simulink model "ThreePhTrans"  (R2020b)
settings: Solver=ode23t  StartTime=0.0  StopTime=0.2  RelTol=1e-3
libraries: powerlib x32
settings Model: Creator=ashka  LastModifiedBy=ashka

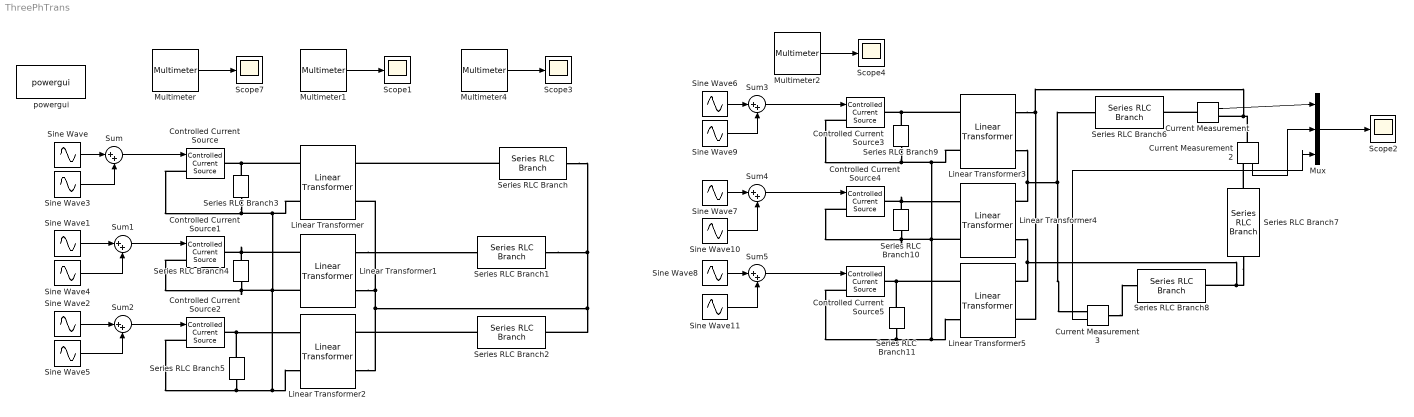
== system ThreePhTrans ==
  Controlled Current Source{,1..5} (6 alike) : powerlib/Electrical Sources/Controlled Current Source  Initialize=on  Source_Type=AC  Amplitude=0  Phase=0  Frequency=0  Measurements=Current
  Current Measurement : powerlib/Measurements/Current Measurement  PhasorSimulation=off  OutputType=Complex  PSBequivalent=0
  Current Measurement2 : powerlib/Measurements/Current Measurement  PhasorSimulation=off  OutputType=Complex  PSBequivalent=0
  Current Measurement3 : powerlib/Measurements/Current Measurement  PhasorSimulation=off  OutputType=Complex  PSBequivalent=0
  Linear Transformer{,1..5} (6 alike) : powerlib/Elements/Linear Transformer  UNITS=SI  NominalPower=[ 10e3 50 ]  winding1=[400 2 0.45856]  winding2=[4000 0.7938 0.084225]  ThreeWindings=off  winding3=[3.15e+05 0.7938 0.084225]  RmLm=[1.0805e+06 2866]  Measurements=None  DataType=on
  Multimeter : powerlib/Measurements/Multimeter  Tag=PoWeRsYsTeMmEaSuReMeNt  PhasorSimulation=off  OutputType=Magnitude  sel=[10 11 12]  L=15  Gain=[1 1 1]  yselected={'Isrc: Controlled Current Source','Isrc: Controlled Current Source1','Isrc: Controlled Current Source2'};  PSBOutputType=1  PSBequivalent=0  AxesSetting=[0,0.1,-100,100]  Display=0  SavedBlockNames=-11
      settings: AttributesFormatString=\n
  Multimeter1 : powerlib/Measurements/Multimeter  Tag=PoWeRsYsTeMmEaSuReMeNt  PhasorSimulation=off  OutputType=Magnitude  sel=[7 8 9]  L=15  Gain=[1 1 1]  yselected={'Ib: Series RLC Branch','Ib: Series RLC Branch1','Ib: Series RLC Branch2'};  PSBOutputType=1  PSBequivalent=0  AxesSetting=[0,0.1,-100,100]  Display=0  SavedBlockNames=-11
      settings: AttributesFormatString=\n
  Multimeter2 : powerlib/Measurements/Multimeter  Tag=PoWeRsYsTeMmEaSuReMeNt  PhasorSimulation=off  OutputType=Magnitude  sel=[13 14 15]  L=15  Gain=[1 1 1]  yselected={'Isrc: Controlled Current Source3','Isrc: Controlled Current Source4','Isrc: Controlled Current Source5'};  PSBOutputType=1  PSBequivalent=0  AxesSetting=[0,0.1,-100,100]  Display=0  SavedBlockNames=-11
      settings: AttributesFormatString=\n
  Multimeter4 : powerlib/Measurements/Multimeter  Tag=PoWeRsYsTeMmEaSuReMeNt  PhasorSimulation=off  OutputType=Magnitude  sel=[1 2 5]  L=15  Gain=[1 1 1]  yselected={'Ub: Series RLC Branch','Ub: Series RLC Branch1','Ub: Series RLC Branch2'};  PSBOutputType=1  PSBequivalent=0  AxesSetting=[0,0.1,-100,100]  Display=0  SavedBlockNames=-11
      settings: AttributesFormatString=\n
  Mux : Mux  Inputs=3
  Scope{1..4,7} (5 alike) : Scope
  Series RLC Branch : powerlib/Elements/Series RLC Branch  LConnTagsString=__new0  RConnTagsString=__new0  BranchType=R  Resistance=100  Inductance=1e-3  SetiL0=off  InitialCurrent=0  Capacitance=1e-6  Setx0=off  InitialVoltage=0  Measurements=Branch voltage and current
  Series RLC Branch1 : powerlib/Elements/Series RLC Branch  LConnTagsString=__new0  RConnTagsString=__new0  BranchType=R  Resistance=100  Inductance=1e-3  SetiL0=off  InitialCurrent=0  Capacitance=1e-6  Setx0=off  InitialVoltage=0  Measurements=Branch voltage and current
  Series RLC Branch10 : powerlib/Elements/Series RLC Branch  LConnTagsString=__new0  RConnTagsString=__new0  BranchType=R  Resistance=1e6  Inductance=1e-3  SetiL0=off  InitialCurrent=0  Capacitance=1e-6  Setx0=off  InitialVoltage=0  Measurements=Branch voltage
  Series RLC Branch11 : powerlib/Elements/Series RLC Branch  LConnTagsString=__new0  RConnTagsString=__new0  BranchType=R  Resistance=1e6  Inductance=1e-3  SetiL0=off  InitialCurrent=0  Capacitance=1e-6  Setx0=off  InitialVoltage=0  Measurements=Branch voltage
  Series RLC Branch2 : powerlib/Elements/Series RLC Branch  LConnTagsString=__new0  RConnTagsString=__new0  BranchType=R  Resistance=100  Inductance=1e-3  SetiL0=off  InitialCurrent=0  Capacitance=1e-6  Setx0=off  InitialVoltage=0  Measurements=Branch voltage and current
  Series RLC Branch3 : powerlib/Elements/Series RLC Branch  LConnTagsString=__new0  RConnTagsString=__new0  BranchType=R  Resistance=1e6  Inductance=1e-3  SetiL0=off  InitialCurrent=0  Capacitance=1e-6  Setx0=off  InitialVoltage=0  Measurements=None
  Series RLC Branch4 : powerlib/Elements/Series RLC Branch  LConnTagsString=__new0  RConnTagsString=__new0  BranchType=R  Resistance=1e6  Inductance=1e-3  SetiL0=off  InitialCurrent=0  Capacitance=1e-6  Setx0=off  InitialVoltage=0  Measurements=None
  Series RLC Branch5 : powerlib/Elements/Series RLC Branch  LConnTagsString=__new0  RConnTagsString=__new0  BranchType=R  Resistance=1e6  Inductance=1e-3  SetiL0=off  InitialCurrent=0  Capacitance=1e-6  Setx0=off  InitialVoltage=0  Measurements=None
  Series RLC Branch6 : powerlib/Elements/Series RLC Branch  LConnTagsString=__new0  RConnTagsString=__new0  BranchType=R  Resistance=100  Inductance=1e-3  SetiL0=off  InitialCurrent=0  Capacitance=1e-6  Setx0=off  InitialVoltage=0  Measurements=None
  Series RLC Branch7 : powerlib/Elements/Series RLC Branch  LConnTagsString=__new0  RConnTagsString=__new0  BranchType=R  Resistance=100  Inductance=1e-3  SetiL0=off  InitialCurrent=0  Capacitance=1e-6  Setx0=off  InitialVoltage=0  Measurements=None
  Series RLC Branch8 : powerlib/Elements/Series RLC Branch  LConnTagsString=__new0  RConnTagsString=__new0  BranchType=R  Resistance=100  Inductance=1e-3  SetiL0=off  InitialCurrent=0  Capacitance=1e-6  Setx0=off  InitialVoltage=0  Measurements=None
  Series RLC Branch9 : powerlib/Elements/Series RLC Branch  LConnTagsString=__new0  RConnTagsString=__new0  BranchType=R  Resistance=1e6  Inductance=1e-3  SetiL0=off  InitialCurrent=0  Capacitance=1e-6  Setx0=off  InitialVoltage=0  Measurements=Branch voltage
  Sine Wave : Sin  Amplitude=40  Frequency=2*pi*50  SampleTime=0
  Sine Wave1 : Sin  Amplitude=40  Frequency=2*pi*50  Phase=120*pi/180  SampleTime=0
  Sine Wave10 : Sin  Amplitude=10  Frequency=2*pi*150  Phase=120*pi/180*30  SampleTime=0
  Sine Wave11 : Sin  Amplitude=10  Frequency=2*pi*150  Phase=240*pi/180*3  SampleTime=0
  Sine Wave2 : Sin  Amplitude=40  Frequency=2*pi*50  Phase=240*pi/180  SampleTime=0
  Sine Wave3 : Sin  Amplitude=10  Frequency=2*pi*150  SampleTime=0
  Sine Wave4 : Sin  Amplitude=10  Frequency=2*pi*150  Phase=120*pi/180*30  SampleTime=0
  Sine Wave5 : Sin  Amplitude=10  Frequency=2*pi*150  Phase=240*pi/180*3  SampleTime=0
  Sine Wave6 : Sin  Amplitude=40  Frequency=2*pi*50  SampleTime=0
  Sine Wave7 : Sin  Amplitude=40  Frequency=2*pi*50  Phase=120*pi/180  SampleTime=0
  Sine Wave8 : Sin  Amplitude=40  Frequency=2*pi*50  Phase=240*pi/180  SampleTime=0
  Sine Wave9 : Sin  Amplitude=10  Frequency=2*pi*150  SampleTime=0
  Sum{,1..5} (6 alike) : Sum  Inputs=|++
  powergui : powerlib/powergui  Priority=1  SimulationMode=Continuous  SampleTime=50e-6  frequency=60  Iterations=50  frequencyindice=0  Pbase=100e6  ErrMax=1e-4  UnitsV=kV  UnitsW=MW  buscounter=0  FunctionMessages=off  echomessages=off  EnableUseOfTLC=off  CurrentSourceSwitches=off  DisableSnubberDevices=off  DisableRonSwitches=off  DisableVfSwitches=off  DisplayEquations=off  AutomaticDiscreteSolvers=off  SolverType=Tustin/Backward Euler (TBE)  Interpol=off  ExternalGateDelay=off  methode=off  Ts=100  x0status=blocks  SPID=on  SwTol=0  HookPort=off  NonlinearTolerance=1e-4  nMaxIteration=100  ContinueOnMaxIteration=off  RestoreLinks=warning  ResistiveCurrentMeasurement=off  Frange=[0:2:500]  Ylog=off  Xlog=on  ShowGrid=off  save=off  variable=ZData  structure=0  ZoomFFT=off  StartTime=0.0  cycles=1  DisplayStyle=1  fundamental=60  FreqAxis=off  MaxFrequency=1000  frequencyindicesteady=1  RmsSteady=1  display=off
  wires:
  Sum/1 -> Controlled Current Source/1
  Sum1/1 -> Controlled Current Source1/1
  Sum2/1 -> Controlled Current Source2/1
  Sine Wave/1 -> Sum/1
  Sine Wave1/1 -> Sum1/1
  Sine Wave2/1 -> Sum2/1
  Sine Wave3/1 -> Sum/2
  Sine Wave4/1 -> Sum1/2
  Sine Wave5/1 -> Sum2/2
  Sum3/1 -> Controlled Current Source3/1
  Sine Wave9/1 -> Sum3/2
  Sine Wave6/1 -> Sum3/1
  Sum5/1 -> Controlled Current Source5/1
  Sum4/1 -> Controlled Current Source4/1
  Sine Wave10/1 -> Sum4/2
  Sine Wave7/1 -> Sum4/1
  Sine Wave8/1 -> Sum5/1
  Sine Wave11/1 -> Sum5/2
  Multimeter/1 -> Scope7/1
  Multimeter1/1 -> Scope1/1
  Multimeter2/1 -> Scope4/1
  Multimeter4/1 -> Scope3/1
  Current Measurement/1 -> Mux/1
  Current Measurement2/1 -> Mux/2
  Current Measurement3/1 -> Mux/3
  Mux/1 -> Scope2/1
  connections:
  Series RLC Branch3/LConn1 -- Linear Transformer/LConn1 -- Controlled Current Source/RConn1
  Series RLC Branch4/LConn1 -- Controlled Current Source1/RConn1 -- Linear Transformer1/LConn1
  Series RLC Branch5/LConn1 -- Linear Transformer2/LConn1 -- Controlled Current Source2/RConn1
  Controlled Current Source2/LConn1 -- Series RLC Branch5/RConn1 -- Linear Transformer1/LConn2 -- Linear Transformer/LConn2 -- Series RLC Branch3/RConn1 -- Controlled Current Source/LConn1 -- Series RLC Branch4/RConn1 -- Controlled Current Source1/LConn1 -- Linear Transformer2/LConn2
  Series RLC Branch/LConn1 -- Linear Transformer/RConn1
  Linear Transformer1/RConn1 -- Series RLC Branch1/LConn1
  Series RLC Branch2/LConn1 -- Linear Transformer2/RConn1
  Linear Transformer2/RConn2 -- Series RLC Branch2/RConn1 -- Series RLC Branch/RConn1 -- Series RLC Branch1/RConn1 -- Linear Transformer1/RConn2 -- Linear Transformer/RConn2
  Series RLC Branch9/RConn1 -- Linear Transformer3/LConn2 -- Series RLC Branch11/RConn1 -- Controlled Current Source5/LConn1 -- Linear Transformer5/LConn2 -- Series RLC Branch10/RConn1 -- Controlled Current Source4/LConn1 -- Linear Transformer4/LConn2 -- Controlled Current Source3/LConn1
  Series RLC Branch11/LConn1 -- Linear Transformer5/LConn1 -- Controlled Current Source5/RConn1
  Series RLC Branch9/LConn1 -- Linear Transformer3/LConn1 -- Controlled Current Source3/RConn1
  Linear Transformer3/RConn2 -- Current Measurement3/RConn1 -- Series RLC Branch6/LConn1 -- Linear Transformer4/RConn1
  Series RLC Branch10/LConn1 -- Controlled Current Source4/RConn1 -- Linear Transformer4/LConn1
  Current Measurement/LConn1 -- Series RLC Branch6/RConn1
  Linear Transformer4/RConn2 -- Series RLC Branch8/RConn1 -- Series RLC Branch7/RConn1 -- Linear Transformer5/RConn1
  Series RLC Branch7/LConn1 -- Current Measurement2/RConn1
  Current Measurement3/LConn1 -- Series RLC Branch8/LConn1
  Linear Transformer5/RConn2 -- Linear Transformer3/RConn1 -- Current Measurement2/LConn1 -- Current Measurement/RConn1
